simulink library "mec_pointmass_generic_ATvoith_DIWA_NXT"  (R2016a)
settings: Solver=ode45  SolverMode=SingleTasking  StartTime=0.0  StopTime=10.0  RelTol=1e-3
undefined symbols (not defined in the file): sMP
(part 3 of 4)

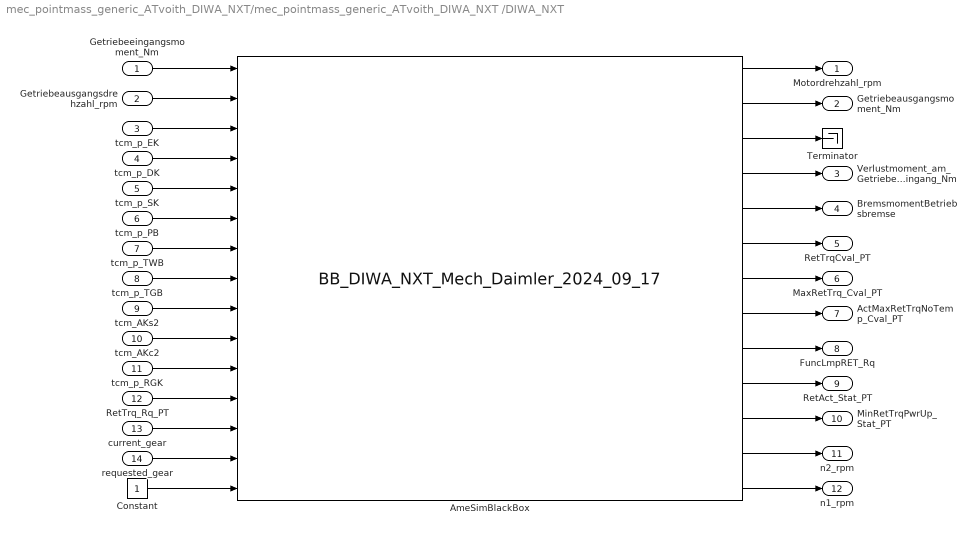
== system mec_pointmass_generic_ATvoith_DIWA_NXT/mec_pointmass_generic_ATvoith_DIWA_NXT /DIWA_NXT ==
  Getriebeeingangsmoment_Nm : Inport
  Getriebeausgangsdrehzahl_rpm : Inport  Port=2
  tcm_p_EK : Inport  Port=3
  tcm_p_DK : Inport  Port=4
  tcm_p_SK : Inport  Port=5
  tcm_p_PB : Inport  Port=6
  tcm_p_TWB : Inport  Port=7
  tcm_p_TGB : Inport  Port=8
  tcm_AKs2 : Inport  Port=9
  tcm_AKc2 : Inport  Port=10
  tcm_p_RGK : Inport  Port=11
  RetTrq_Rq_PT : Inport  Port=12
  current_gear : Inport  Port=13
  requested_gear : Inport  Port=14
  AmeSimBlackBox : S-Function  FunctionName=BB_DIWA_NXT_Mech_Daimler_2024_09_17  Parameters=[1 0.01],DIWA_BB_ParNames,DIWA_BB_ParValues  SFunctionDeploymentMode=off  EnableBusSupport=off
      mask Display:
      | disp('LMS Amesim black-box:\nBB_DIWA_NXT_Mech_Daimler_2024_09_17');
      | port_label('input',1,'Getriebeeingangsmoment_Nm');
      | port_label('input',2,'Getriebeausgangsdrehzahl_rpm');
      | port_label('input',3,'p_EK');
      | port_label('input',4,'p_DK');
      | port_label('input',5,'p_SK');
      | port_label('input',6,'p_PB');
      | port_label('input',7,'p_TWB');
      | port_label('input',8,'p_TGB');
      | port_label('input',9,'Direktgangklaue_AKs2');
      | port_label('input',10,'Schnellgangklaue_AKc2');
      | port_label('input',11,'p_RGK');
      | port_label('input',12,'RetTrq_Rq_PT');
      | port_label('input',13,'current_gear');
      | port_label('input',14,'requested_gear');
      | port_label('input',15,'StartStop');
      | 
      | 
      | 
      | port_label('output',1,'Motordrehzahl_rpm');
      | port_label('output',2,'Getriebeausgangsmoment_Nm');
      | port_label('output',3,'Summentraegheitsmoment_kgm2');
      | port_label('output',4,'Verlustmoment_am_Getriebeeingang_Nm');
      | port_label('output',5,'BremsmomentBetriebsbremse');
      | port_label('output',6,'RetTrq_Cval_PT');
      | port_label('output',7,'MaxRetTrq_Cval_PT');
      | port_label('output',8,'ActMaxRetTrqNoTemp_Cval_PT');
      | port_label('output',9,'FuncLmpRET_Rq');
      | port_label('output',10,'RetActv_Stat_PT');
      | port_label('output',11,'MinRetTrqPwrUp_Stat_PT');
      | port_label('output',12,'n2_rpm');
      | port_label('output',13,'n1_rpm');
  Constant : Constant
  Terminator : Terminator
  Motordrehzahl_rpm : Outport
  Getriebeausgangsmoment_Nm : Outport  Port=2
  Verlustmoment_am_Getriebeeingang_Nm : Outport  Port=3
  BremsmomentBetriebsbremse : Outport  Port=4
  RetTrqCval_PT : Outport  Port=5
  MaxRetTrq_Cval_PT : Outport  Port=6
  ActMaxRetTrqNoTemp_Cval_PT : Outport  Port=7
  FuncLmpRET_Rq : Outport  Port=8
  RetAct_Stat_PT : Outport  Port=9
  MinRetTrqPwrUp_Stat_PT : Outport  Port=10
  n2_rpm : Outport  Port=11
  n1_rpm : Outport  Port=12
  wires:
  tcm_p_EK/1 -> AmeSimBlackBox/3
  tcm_p_DK/1 -> AmeSimBlackBox/4
  tcm_p_SK/1 -> AmeSimBlackBox/5
  tcm_p_PB/1 -> AmeSimBlackBox/6
  tcm_p_TWB/1 -> AmeSimBlackBox/7
  tcm_p_TGB/1 -> AmeSimBlackBox/8
  tcm_AKs2/1 -> AmeSimBlackBox/9
  tcm_AKc2/1 -> AmeSimBlackBox/10
  Getriebeeingangsmoment_Nm/1 -> AmeSimBlackBox/1
  AmeSimBlackBox/1 -> Motordrehzahl_rpm/1
  Getriebeausgangsdrehzahl_rpm/1 -> AmeSimBlackBox/2
  AmeSimBlackBox/2 -> Getriebeausgangsmoment_Nm/1
  AmeSimBlackBox/3 -> Terminator/1
  AmeSimBlackBox/4 -> Verlustmoment_am_Getriebeeingang_Nm/1
  AmeSimBlackBox/5 -> BremsmomentBetriebsbremse/1
  AmeSimBlackBox/6 -> RetTrqCval_PT/1
  tcm_p_RGK/1 -> AmeSimBlackBox/11
  RetTrq_Rq_PT/1 -> AmeSimBlackBox/12
  Constant/1 -> AmeSimBlackBox/15
  AmeSimBlackBox/7 -> MaxRetTrq_Cval_PT/1
  AmeSimBlackBox/8 -> ActMaxRetTrqNoTemp_Cval_PT/1
  AmeSimBlackBox/9 -> FuncLmpRET_Rq/1
  AmeSimBlackBox/10 -> RetAct_Stat_PT/1
  AmeSimBlackBox/11 -> MinRetTrqPwrUp_Stat_PT/1
  AmeSimBlackBox/12 -> n2_rpm/1
  AmeSimBlackBox/13 -> n1_rpm/1
  requested_gear/1 -> AmeSimBlackBox/14
  current_gear/1 -> AmeSimBlackBox/13

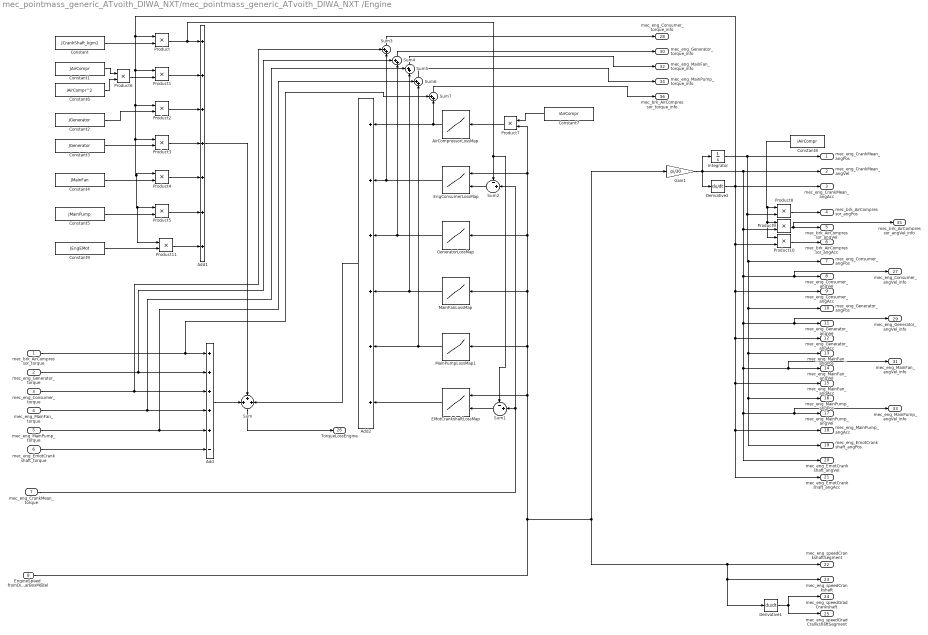
== system mec_pointmass_generic_ATvoith_DIWA_NXT/mec_pointmass_generic_ATvoith_DIWA_NXT /Engine ==
  mec_brk_AirCompressor_torque : Inport
  mec_eng_Generator_torque : Inport  Port=2
  mec_eng_Consumer_torque : Inport  Port=3
  mec_eng_MainFan_torque : Inport  Port=4
  mec_eng_MainPump_torque : Inport  Port=5
  mec_eng_EmotCrankshaft_torque : Inport  Port=6
  mec_eng_CrankMean_torque : Inport  Port=7
  EngineSpeed_fromDiwaGearBoxModel : Inport  Port=8
  Add : Sum  Inputs=+++++-
  Add1 : Sum  Inputs=+++++++
  Add2 : Sum  Inputs=++++++
  AirCompressorLossMap : Lookup_n-D  NumberOfTableDimensions=1  BreakpointsForDimension1=airComprLoss_x_speed_rpm  Table=airComprLoss_map_lossTorque_Nm  InternalRulePriority=Speed  RndMeth=Simplest  InputSameDT=on
  Constant : Constant  Value=JCrankShaft_kgm2
  Constant1 : Constant  Value=JAirCompr
  Constant2 : Constant  Value=JGenerator
  Constant3 : Constant  Value=JGenerator
  Constant4 : Constant  Value=JMainFan
  Constant5 : Constant  Value=JMainPump
  Constant6 : Constant  Value=iAirCompr^2
  Constant7 : Constant  Value=iAirCompr
  Constant8 : Constant  Value=iAirCompr
  Constant9 : Constant  Value=JEngEMot
  Derivative1 : Derivative
  Derivative2 : Derivative
  EMotCrankshaftLossMap : Lookup_n-D  BreakpointsForDimension1=engEMotLoss_x_speed_rpm  BreakpointsForDimension2=engEMotLoss_y_torque_Nm  Table=engEMotLoss_map_lossTorque_Nm  InternalRulePriority=Speed  RndMeth=Simplest  InputSameDT=on
  EngConsumerLossMap : Lookup_n-D  BreakpointsForDimension1=engConsumerLoss_x_speed_rpm  BreakpointsForDimension2=engConsumerLoss_y_torque_Nm  Table=engConsumerLoss_map_lossTorque_Nm  InternalRulePriority=Speed  RndMeth=Simplest  InputSameDT=on
  Gain1 : Gain  Gain=pi/30
  GeneratorLossMap : Lookup_n-D  NumberOfTableDimensions=1  BreakpointsForDimension1=generatorLoss_x_speed_rpm  Table=generatorLoss_map_lossTorque_Nm  InternalRulePriority=Speed  RndMeth=Simplest  InputSameDT=on
  Integrator : Integrator
  MainFanLossMap : Lookup_n-D  NumberOfTableDimensions=1  BreakpointsForDimension1=mainFanLoss_x_speed_rpm  Table=mainFanLoss_map_lossTorque_Nm  InternalRulePriority=Speed  RndMeth=Simplest  InputSameDT=on
  MainPumpLossMap1 : Lookup_n-D  NumberOfTableDimensions=1  BreakpointsForDimension1=mainPumpLoss_x_speed_rpm  Table=mainPumpLoss_map_lossTorque_Nm  InternalRulePriority=Speed  RndMeth=Simplest  InputSameDT=on
  Product{,1..11} (12 alike) : Product
  Sum : Sum  Inputs=+++
  Sum1 : Sum  Inputs=-+|
  Sum2 : Sum  Inputs=-+|
  Sum{3..7} (5 alike) : Sum  Inputs=++|
  mec_eng_CrankMean_angPos : Outport
  mec_eng_CrankMean_angVel : Outport  Port=2
  mec_eng_CrankMean_angAcc : Outport  Port=3
  mec_brk_AirCompressor_angPos : Outport  Port=4
  mec_brk_AirCompressor_angVel : Outport  Port=5
  mec_brk_AirCompressor_angAcc : Outport  Port=6
  mec_eng_Consumer_angPos : Outport  Port=7
  mec_eng_Consumer_angVel : Outport  Port=8
  mec_eng_Consumer_angAcc : Outport  Port=9
  mec_eng_Generator_angPos : Outport  Port=10
  mec_eng_Generator_angVel : Outport  Port=11
  mec_eng_Generator_angAcc : Outport  Port=12
  mec_eng_MainFan_angPos : Outport  Port=13
  mec_eng_MainFan_angVel : Outport  Port=14
  mec_eng_MainFan_angAcc : Outport  Port=15
  mec_eng_MainPump_angPos : Outport  Port=16
  mec_eng_MainPump_angVel : Outport  Port=17
  mec_eng_MainPump_angAcc : Outport  Port=18
  mec_eng_EmotCrankshaft_angPos : Outport  Port=19
  mec_eng_EmotCrankshaft_angVel : Outport  Port=20
  mec_eng_EmotCrankshaft_angAcc : Outport  Port=21
  mec_eng_speedCrankshaftSegment : Outport  Port=22
  mec_eng_speedCrankshaft : Outport  Port=23
  mec_eng_speedGradCrankshaft : Outport  Port=24
  mec_eng_speedGradCrankshaftSegment : Outport  Port=25
  TorqueLossEngine : Outport  Port=26
  mec_eng_Consumer_angVel_info : Outport  Port=27
  mec_eng_Consumer_torque_info : Outport  Port=28
  mec_eng_Generator_angVel_info : Outport  Port=29
  mec_eng_Generator_torque_info : Outport  Port=30
  mec_eng_MainFan_angVel_info : Outport  Port=31
  mec_eng_MainFan_torque_info : Outport  Port=32
  mec_eng_MainPump_angVel_info : Outport  Port=33
  mec_eng_MainPump_torque_info : Outport  Port=34
  mec_brk_AirCompressor_angVel_info : Outport  Port=35
  mec_brk_AirCompressor_torque_info : Outport  Port=36
  wires:
  mec_eng_MainPump_torque/1 -> Sum6/1, Add/5
  mec_eng_MainFan_torque/1 -> Sum5/1, Add/4
  Constant1/1 -> Product6/1
  Constant2/1 -> Product2/2
  Constant4/1 -> Product4/2
  Constant3/1 -> Product3/2
  Constant5/1 -> Product5/2
  Constant/1 -> Product/2
  mec_brk_AirCompressor_torque/1 -> Sum7/1, Add/1
  mec_eng_Generator_torque/1 -> Sum4/1, Add/2
  Constant6/1 -> Product6/2
  AirCompressorLossMap/1 -> Sum7/2, Add2/1
  Product7/1 -> AirCompressorLossMap/1
  Sum/1 -> TorqueLossEngine/1
  Product2/1 -> Add1/3
  Product/1 -> Sum1/1, Sum2/1, Add1/1
  Product3/1 -> Add1/4
  Constant7/1 -> Product7/1
  Sum2/1 -> EngConsumerLossMap/2
  Product1/1 -> Add1/2
  Product4/1 -> Add1/5
  Add/1 -> Sum/1
  Add2/1 -> Sum/3
  Product6/1 -> Product1/2
  Add1/1 -> Sum/2
  MainFanLossMap/1 -> Add2/4, Sum5/2
  Product5/1 -> Add1/6
  MainPumpLossMap1/1 -> Sum6/2, Add2/5
  mec_eng_CrankMean_torque/1 -> Sum2/2, Sum1/2
  Derivative1/1 -> mec_eng_speedGradCrankshaft/1, mec_eng_speedGradCrankshaftSegment/1
  Product8/1 -> mec_brk_AirCompressor_angPos/1
  Constant8/1 -> Product10/1, Product9/1, Product8/1
  Product9/1 -> mec_brk_AirCompressor_angVel/1, mec_brk_AirCompressor_angVel_info/1
  Product10/1 -> mec_brk_AirCompressor_angAcc/1
  Derivative2/1 -> mec_eng_EmotCrankshaft_angAcc/1, mec_eng_MainPump_angAcc/1, mec_eng_MainFan_angAcc/1, mec_eng_Generator_angAcc/1, mec_eng_Consumer_angAcc/1, Product10/2, Product/1, Product11/1, Product5/1, Product4/1, Product3/1, Product2/1, Product1/1, mec_eng_CrankMean_angAcc/1
  Integrator/1 -> mec_eng_EmotCrankshaft_angPos/1, mec_eng_MainPump_angPos/1, mec_eng_MainFan_angPos/1, mec_eng_Generator_angPos/1, mec_eng_Consumer_angPos/1, Product8/2, mec_eng_CrankMean_angPos/1
  Gain1/1 -> mec_eng_EmotCrankshaft_angVel/1, mec_eng_MainPump_angVel/1, mec_eng_MainPump_angVel_info/1, mec_eng_MainFan_angVel_info/1, mec_eng_MainFan_angVel/1, mec_eng_Generator_angVel/1, mec_eng_Generator_angVel_info/1, mec_eng_Consumer_angVel/1, mec_eng_Consumer_angVel_info/1, Product9/2, mec_eng_CrankMean_angVel/1, Integrator/1, Derivative2/1
  Constant9/1 -> Product11/2
  Product11/1 -> Add1/7
  EMotCrankshaftLossMap/1 -> Add2/6
  Sum1/1 -> EMotCrankshaftLossMap/2
  EngineSpeed_fromDiwaGearBoxModel/1 -> Gain1/1, Derivative1/1, mec_eng_speedCrankshaft/1, mec_eng_speedCrankshaftSegment/1, EMotCrankshaftLossMap/1, Product7/2, EngConsumerLossMap/1, GeneratorLossMap/1, MainFanLossMap/1, MainPumpLossMap1/1
  mec_eng_EmotCrankshaft_torque/1 -> Add/6
  Sum3/1 -> mec_eng_Consumer_torque_info/1
  EngConsumerLossMap/1 -> Add2/2, Sum3/2
  mec_eng_Consumer_torque/1 -> Sum3/1, Add/3
  Sum4/1 -> mec_eng_Generator_torque_info/1
  GeneratorLossMap/1 -> Sum4/2, Add2/3
  Sum5/1 -> mec_eng_MainFan_torque_info/1
  Sum6/1 -> mec_eng_MainPump_torque_info/1
  Sum7/1 -> mec_brk_AirCompressor_torque_info/1
